simulink model "psbacvoltage"  (Simulink 6.0)
settings: Solver=VariableStepDiscrete  SolverMode=SingleTasking  StartTime=0.0  StopTime=888  MaxStep=1e-03  RelTol=1e-3  AbsTol=1e-6
libraries: powerlib2 x4
settings Model: Creator=patrice  LastModifiedBy=batserve  ExtModeTrigMode=oneshot  ExtModeArmWhenConnect=off  ExtModeAutoUpdateStatusClock=off
settings DataIOCC: LimitDataPoints=off
settings OptimizationCC: BooleanDataType=off
settings DebuggingCC: SolverPrmCheckMsg=none
settings HardwareCC: TargetUnknown=on
settings RTWCC: TemplateMakefile=grt_unix.tmf

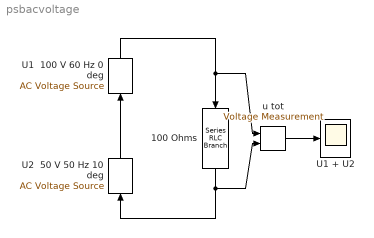
== system psbacvoltage ==
  100 Ohms : powerlib2/Elements/Series RLC Branch  Tag=PoWeRsYsTeMbLoCk  Orientation=down  a=100  b=0  c=inf  mesure=None  PSBOutputType=1
  U1  100 V 60 Hz 0 deg : powerlib2/Electrical Sources/AC Voltage Source  Tag=PoWeRsYsTeMbLoCk  Orientation=up  A=100  P=0  F=60  stime=0  mesure=None  PSBOutputType=1
  U1 + U2 : Scope
      settings: TickLabels=on  TimeRange=0.5  YMin=-180  YMax=180  DataFormat=Array
  U2  50 V 50 Hz 10 deg : powerlib2/Electrical Sources/AC Voltage Source  Tag=PoWeRsYsTeMbLoCk  Orientation=up  A=50  P=10  F=50  stime=0  mesure=None  PSBOutputType=1
  u tot : powerlib2/Measurements/Voltage Measurement  Tag=PoWeRsYsTeMmEaSuReMeNt  PSBOutputType=0  PSBequivalent=1
  wires:
  U2  50 V 50 Hz 10 deg/1 -> U1  100 V 60 Hz 0 deg/1
  100 Ohms/1 -> U2  50 V 50 Hz 10 deg/1, u tot/2
  U1  100 V 60 Hz 0 deg/1 -> 100 Ohms/1, u tot/1
  u tot/1 -> U1 + U2/1
